simulink model "sim_battery_system"  (R2018b)
settings: Solver=FixedStepDiscrete  StartTime=0.0  StopTime=SimPara.t_sim  FixedStep=SimPara.t_step  RelTol=1e-3
undefined symbols (not defined in the file or in its folder): A, BatPara, i, LSAPara, p, SimPara, SysPara, x2_cal, x3_cal, x_cal
libraries: simulink x14, dspstat3 x4, dspindex x1
(part 2 of 4)

== system sim_battery_system/Battery system simulation/Thermal Submodel/Cell heat transport and heat dissipation ==
  PQ_cell : Inport
  BatPara : Inport  Port=2
  T_cell_in : Inport  Port=3
  alpha_cell_ambient : Inport  Port=4
  T_cell_ambient : Inport  Port=5
  Enable : EnablePort
  Heat dissipation model : Subsystem
  Heat transfer between cells : Subsystem  Variant=on
  Lumped mass thermal cell model : Subsystem  VariantControl=SimPara.heat_exchange_enable == 0
  T_cell [°C] : Outport  InitialOutput=SysPara.BatStateInit.thermal.T_cell
  PQ_ambient [W] : Outport  Port=2  InitialOutput=0
  PQ_transfer [W] : Outport  Port=3  InitialOutput=0
  wires:
  Lumped mass thermal cell model/1(T_cell [°C]) -> T_cell [°C]/1
  PQ_cell/1 -> Lumped mass thermal cell model/1(PQ_cell)
  BatPara/1 -> Heat dissipation model/2(BatPara), Lumped mass thermal cell model/2(BatPara)
  T_cell_in/1 -> Heat transfer between cells/1(T_cell_in), Heat dissipation model/1(T_cells_in), Lumped mass thermal cell model/3(T_cell_in)
  T_cell_ambient/1 -> Heat dissipation model/3(T_cell_ambient)
  alpha_cell_ambient/1 -> Heat dissipation model/4(alpha_cell_ambient)
  Heat dissipation model/1(PQ_ambient) -> PQ_ambient [W]/1, Lumped mass thermal cell model/4(PQ_ambient)
  Heat transfer between cells/1(PQ_transfer) -> PQ_transfer [W]/1, Lumped mass thermal cell model/5(PQ_transfer)

== system sim_battery_system/Battery system simulation/Thermal Submodel/Irreversible heat generation ==
  note: Calculation of ohmic/irreversible heat losses:
      |
      | -> Equation PQ_Cells,irr = R_Cells,total * I_Cells^2
      | -> R_Cells is the sum of all voltage drops in the cell (internal resistance and RC-Elements)
  U_R [V] : Inport
  U_RC : Inport  Port=2
  I_Cells [A] : Inport  Port=3
  Abs : Abs
  Add : Sum
  Bus Selector : BusSelector  OutputSignals=sum_U_RC [V]
  Product : Product  Inputs=**  RndMeth=Zero
  PQ_cell,irr [W] : Outport
  wires:
  I_Cells [A]/1 -> Product/2
  Add/1 -> Product/1
  Product/1 -> Abs/1
  U_R [V]/1 -> Add/1
  U_RC/1 -> Bus Selector/1
  Abs/1 -> PQ_cell,irr [W]/1  "PQ_cell,irr"
  Bus Selector/1 -> Add/2  "<sum_U_RC [V]>"

== system sim_battery_system/Battery system simulation/Thermal Submodel/Reversible heat generation ==
  note: Calculation of reversible heat losses in the cells
      |
      | PQ_Cells,rev = - I_cell * T_cell * (dUocv/dT_cell) = - I_cell * T_cell * EnCo
      |
      | Eddahech et al., 2013 - Thermal characterization of a high-power lithium-ion battery
  I_Cells [A] : Inport
  T_Cells [°C] : Inport  Port=2
  BatPara : Inport  Port=3
  Bus Selector : BusSelector  OutputSignals=thermal.EnCo
  Gain : Gain  Gain=-1
  Product : Product  Inputs=***  RndMeth=Zero
  PQ_cell,rev [W] : Outport
  wires:
  BatPara/1 -> Bus Selector/1
  Product/1 -> Gain/1
  T_Cells [°C]/1 -> Product/3
  I_Cells [A]/1 -> Product/1
  Gain/1 -> PQ_cell,rev [W]/1  "PQ_cell,rev"
  Bus Selector/1 -> Product/2  "<EnCo>"

== system sim_battery_system/Monitoring and Logging/Load Spectrum Analysis/Load Spectrum Analysis OFF ==
  BatState_el : Inport
  BatState_th : Inport  Port=2
  BatPara : Inport  Port=3
  Terminator : Terminator
  Terminator1 : Terminator
  Terminator2 : Terminator
  wires:
  BatState_el/1 -> Terminator/1
  BatState_th/1 -> Terminator1/1
  BatPara/1 -> Terminator2/1

== system sim_battery_system/Monitoring and Logging/Load Spectrum Analysis/Load Spectrum Analysis ON ==
  BatState_el : Inport
  BatState_th : Inport  Port=2
  BatPara : Inport  Port=3
  Bus Selector : BusSelector  OutputSignals=SOC,I_cell [A],U_cell [V]
  Bus Selector1 : BusSelector  OutputSignals=T_cell [°C]
  Bus Selector2 : BusSelector  OutputSignals=electrical.C_A [Ah]
  Load Spectrum Analysis ON : Subsystem  VariantControl=SimPara.LoadSpectra == 1
  wires:
  BatState_el/1 -> Bus Selector/1
  BatState_th/1 -> Bus Selector1/1
  BatPara/1 -> Bus Selector2/1
  Bus Selector/1 -> Load Spectrum Analysis ON/1(SOC)  "<SOC>"
  Bus Selector/2 -> Load Spectrum Analysis ON/2(I_cell [A])  "<I_cell [A]>"
  Bus Selector/3 -> Load Spectrum Analysis ON/3(U_Cell [A])  "<U_cell [V]>"
  Bus Selector1/1 -> Load Spectrum Analysis ON/4(T_cell [°C])  "<T_cell [°C]>"
  Bus Selector2/1 -> Load Spectrum Analysis ON/5(C_A [Ah])  "<C_A [Ah]>"

== system sim_battery_system/Monitoring and Logging/Logging of Variables/Calc Temp Gradient ==
  T_cell : Inport
  Abs : Abs
  Add : Sum  Inputs=-+
  MinMax : MinMax
  MinMax1 : MinMax  Function=max
  Reshape : Reshape
  T_cell_gradient : Outport
  wires:
  T_cell/1 -> Reshape/1
  MinMax/1 -> Add/1
  MinMax1/1 -> Add/2
  Add/1 -> Abs/1
  Abs/1 -> T_cell_gradient/1
  Reshape/1 -> MinMax1/1, MinMax/1

== system sim_battery_system/Monitoring and Logging/Temperature Sensor Simulation/Enable//disable temperature sensors ==
  T_cell : Inport
  TempSensors OFF : Subsystem  VariantControl=SimPara.TempSensors_enable==0
  TempSensors ON : Subsystem  VariantControl=SimPara.TempSensors_enable==1
  T_sensors [°C] : Outport

== system sim_battery_system/Monitoring and Logging/Temperature Sensor Simulation/Rebuild bus structure ==
  T_sensors : Inport
  Bat_state_th_in : Inport  Port=2
  Bus Creator1 : BusCreator  Inputs=7
  Bus Selector1 : BusSelector  OutputSignals=PQ_cell [W],T_cell [°C],T_cell_ambient,alpha_cell_ambient,PQ_ambient [W],PQ_transfer [W]
  bat_state_th_out : Outport
  wires:
  Bus Selector1/4 -> Bus Creator1/4  "<alpha_cell_ambient>"
  Bus Selector1/1 -> Bus Creator1/1  "<PQ_cell [W]>"
  Bus Selector1/2 -> Bus Creator1/2  "<T_cell [°C]>"
  T_sensors/1 -> Bus Creator1/7
  Bus Selector1/3 -> Bus Creator1/3  "<T_cell_ambient>"
  Bat_state_th_in/1 -> Bus Selector1/1
  Bus Creator1/1 -> bat_state_th_out/1  "bat_state_th"
  Bus Selector1/5 -> Bus Creator1/5  "<PQ_ambient [W]>"
  Bus Selector1/6 -> Bus Creator1/6  "<PQ_transfer [W]>"

== system sim_battery_system/Battery system simulation/Electrical Submodel/Electric potential (single cell)/Cell ECM RC-element 1 ==
  BatState_In : Inport
  BatPara : Inport  Port=2
  dt [s] : Inport  Port=3
  Enable : EnablePort
  Bus Selector : BusSelector  OutputSignals=U_RC.U_RC1 [V],I_cell [A]
  Bus Selector1 : BusSelector  OutputSignals=electrical.R1 [Ohm],electrical.C1 [F]
  Constant : Constant  VectorParams1D=off
  Gain : Gain  Gain=-1
  Math Function : Math  SaturateOnIntegerOverflow=on
  Product : Product  Inputs=**  RndMeth=Zero
  Product1 : Product  Inputs=/*  RndMeth=Zero
  Product2 : Product  Inputs=***  RndMeth=Zero
  Product3 : Product  Inputs=**  RndMeth=Zero
  Sum : Sum  Inputs=-+
  Sum1 : Sum
  U_RC1 [V] : Outport  OutputWhenDisabled=reset  InitialOutput=zeros(SysPara.p,SysPara.s)
  wires:
  Product/1 -> Product1/1
  Product3/1 -> Sum1/1
  Product1/1 -> Gain/1
  Sum1/1 -> U_RC1 [V]/1
  Gain/1 -> Math Function/1
  Product2/1 -> Sum1/2
  Bus Selector/1 -> Product3/1  "<U_RC1 [V]>"
  Math Function/1 -> Sum/1, Product3/2
  Sum/1 -> Product2/1
  Bus Selector1/1 -> Product2/2, Product/1  "<R1 [Ohm]>"
  BatPara/1 -> Bus Selector1/1
  dt [s]/1 -> Product1/2
  Bus Selector/2 -> Product2/3  "<I_cell [A]>"
  BatState_In/1 -> Bus Selector/1
  Bus Selector1/2 -> Product/2  "<C1 [F]>"
  Constant/1 -> Sum/2

== system sim_battery_system/Battery system simulation/Electrical Submodel/Electric potential (single cell)/Cell ECM RC-element 2 ==
  BatState_In : Inport
  BatPara : Inport  Port=2
  dt [s] : Inport  Port=3
  Enable : EnablePort
  Bus Selector : BusSelector  OutputSignals=U_RC.U_RC2 [V],I_cell [A]
  Bus Selector1 : BusSelector  OutputSignals=electrical.R2 [Ohm],electrical.C2 [F]
  Constant : Constant  VectorParams1D=off
  Gain : Gain  Gain=-1
  Math Function : Math  SaturateOnIntegerOverflow=on
  Product : Product  Inputs=**  RndMeth=Zero
  Product1 : Product  Inputs=/*  RndMeth=Zero
  Product2 : Product  Inputs=***  RndMeth=Zero
  Product3 : Product  Inputs=**  RndMeth=Zero
  Sum : Sum  Inputs=-+
  Sum1 : Sum
  U_RC2 [V] : Outport  OutputWhenDisabled=reset  InitialOutput=zeros(SysPara.p,SysPara.s)
  wires:
  Product/1 -> Product1/1
  Product3/1 -> Sum1/1
  Product1/1 -> Gain/1
  Sum1/1 -> U_RC2 [V]/1
  Gain/1 -> Math Function/1
  Product2/1 -> Sum1/2
  Bus Selector/1 -> Product3/1  "<U_RC2 [V]>"
  Math Function/1 -> Sum/1, Product3/2
  Sum/1 -> Product2/1
  Bus Selector1/1 -> Product2/2, Product/1  "<R2 [Ohm]>"
  BatPara/1 -> Bus Selector1/1
  dt [s]/1 -> Product1/2
  Bus Selector/2 -> Product2/3  "<I_cell [A]>"
  BatState_In/1 -> Bus Selector/1
  Bus Selector1/2 -> Product/2  "<C2 [F]>"
  Constant/1 -> Sum/2

== system sim_battery_system/Battery system simulation/Electrical Submodel/Electric potential (single cell)/Cell ECM RC-element 3 ==
  BatState_In : Inport
  BatPara : Inport  Port=2
  dt [s] : Inport  Port=3
  Enable : EnablePort
  Bus Selector : BusSelector  OutputSignals=U_RC.U_RC3 [V],I_cell [A]
  Bus Selector1 : BusSelector  OutputSignals=electrical.R3 [Ohm],electrical.C3 [F]
  Constant : Constant  VectorParams1D=off
  Gain : Gain  Gain=-1
  Math Function : Math  SaturateOnIntegerOverflow=on
  Product : Product  Inputs=**  RndMeth=Zero
  Product1 : Product  Inputs=/*  RndMeth=Zero
  Product2 : Product  Inputs=***  RndMeth=Zero
  Product3 : Product  Inputs=**  RndMeth=Zero
  Sum : Sum  Inputs=-+
  Sum1 : Sum
  U_RC3 [V] : Outport  OutputWhenDisabled=reset  InitialOutput=zeros(SysPara.p,SysPara.s)
  wires:
  Product/1 -> Product1/1
  Product3/1 -> Sum1/1
  Product1/1 -> Gain/1
  Sum1/1 -> U_RC3 [V]/1
  Gain/1 -> Math Function/1
  Product2/1 -> Sum1/2
  Bus Selector/1 -> Product3/1  "<U_RC3 [V]>"
  Math Function/1 -> Sum/1, Product3/2
  Sum/1 -> Product2/1
  Bus Selector1/1 -> Product2/2, Product/1  "<R3 [Ohm]>"
  BatPara/1 -> Bus Selector1/1
  dt [s]/1 -> Product1/2
  Bus Selector/2 -> Product2/3  "<I_cell [A]>"
  BatState_In/1 -> Bus Selector/1
  Bus Selector1/2 -> Product/2  "<C3 [F]>"
  Constant/1 -> Sum/2

== system sim_battery_system/Battery system simulation/Electrical Submodel/Electric potential (single cell)/Cell ECM RC-element 4 ==
  BatState_In : Inport
  BatPara : Inport  Port=2
  dt [s] : Inport  Port=3
  Enable : EnablePort
  Bus Selector : BusSelector  OutputSignals=U_RC.U_RC4 [V],I_cell [A]
  Bus Selector1 : BusSelector  OutputSignals=electrical.R4 [Ohm],electrical.C4 [F]
  Constant : Constant  VectorParams1D=off
  Gain : Gain  Gain=-1
  Math Function : Math  SaturateOnIntegerOverflow=on
  Product : Product  Inputs=**  RndMeth=Zero
  Product1 : Product  Inputs=/*  RndMeth=Zero
  Product2 : Product  Inputs=***  RndMeth=Zero
  Product3 : Product  Inputs=**  RndMeth=Zero
  Sum : Sum  Inputs=-+
  Sum1 : Sum
  U_RC4 [V] : Outport  OutputWhenDisabled=reset  InitialOutput=zeros(SysPara.p,SysPara.s)
  wires:
  Product/1 -> Product1/1
  Product3/1 -> Sum1/1
  Product1/1 -> Gain/1
  Sum1/1 -> U_RC4 [V]/1
  Gain/1 -> Math Function/1
  Product2/1 -> Sum1/2
  Bus Selector/1 -> Product3/1  "<U_RC4 [V]>"
  Math Function/1 -> Sum/1, Product3/2
  Sum/1 -> Product2/1
  Bus Selector1/1 -> Product2/2, Product/1  "<R4 [Ohm]>"
  BatPara/1 -> Bus Selector1/1
  dt [s]/1 -> Product1/2
  Bus Selector/2 -> Product2/3  "<I_cell [A]>"
  BatState_In/1 -> Bus Selector/1
  Bus Selector1/2 -> Product/2  "<C4 [F]>"
  Constant/1 -> Sum/2

== system sim_battery_system/Battery system simulation/Electrical Submodel/Electric potential (single cell)/Cell Hysteresis Voltage ==
  note: Zugrunde liegende Formel aus "Verbrugge, 2007 - Adaptive, multi-parameter battery state estimator with optimized time weighting factors"
  note: Wenn kein Hysteresemodell verwendet werden soll
      |  beta = 0 setzen
  BatState_In : Inport
  dt [s] : Inport  Port=2
  Add : Sum  Inputs=-+
  Add1 : Sum
  Bus Selector : BusSelector  OutputSignals=U_Hysteresis [V],I_cell [A],SOC
  Product : Product
  Product1 : Product  Inputs=4
  Sign : Signum
  V_H,max(SOC) : Lookup_n-D  NumberOfTableDimensions=1  BreakpointsForDimension1=BatPara.electrical.OCV.SOC  BeginIndexSearchUsingPreviousIndexResult=on  Table=BatPara.electrical.OCV.U_hyst  ExtrapMethod=Clip  DiagnosticForOutOfRangeInput=Warning  RemoveProtectionInput=on  UseLastTableValue=on  InternalRulePriority=Speed  RndMeth=Simplest  InputSameDT=on
  beta : Constant  Value=BatPara.electrical.OCV.beta_hyst  VectorParams1D=off
  U_Hysteresis [V] : Outport
  wires:
  Bus Selector/2 -> Sign/1, Product1/3  "<I_cell [A]>"
  Bus Selector/3 -> V_H,max(SOC)/1  "<SOC>"
  V_H,max(SOC)/1 -> Add/2
  Add/1 -> Product1/4  "V_H,max-sign(I)*V_H"
  dt [s]/1 -> Product1/2
  Product1/1 -> Add1/2
  Add1/1 -> U_Hysteresis [V]/1
  Sign/1 -> Product/2  "sign(I)"
  Product/1 -> Add/1
  BatState_In/1 -> Bus Selector/1
  Bus Selector/1 -> Add1/1, Product/1  "<U_Hysteresis [V]>"
  beta/1 -> Product1/1

== system sim_battery_system/Battery system simulation/Electrical Submodel/Electric potential (single cell)/Cell Open-Circuit-Voltage ==
  SOC [-] : Inport
  BatPara : Inport  Port=2
  SOC --> U : Lookup_n-D  NumberOfTableDimensions=1  BreakpointsForDimension1=BatPara.electrical.OCV.SOC  BreakpointsForDimension2=[1:3]  IndexSearchMethod=Linear search  BeginIndexSearchUsingPreviousIndexResult=on  Table=BatPara.electrical.OCV.U  DiagnosticForOutOfRangeInput=Warning  RemoveProtectionInput=on  RndMeth=Simplest  InputSameDT=on
  Terminator : Terminator
  U_OCV [V] : Outport
  wires:
  SOC [-]/1 -> SOC --> U/1
  SOC --> U/1 -> U_OCV [V]/1
  BatPara/1 -> Terminator/1

== system sim_battery_system/Battery system simulation/Electrical Submodel/Electric potential (single cell)/Cell SOC ==
  BatPara : Inport
  BatState_In : Inport  Port=2
  dt [s] : Inport  Port=3
  Ah in As : Gain  Gain=3600
  Bus Selector : BusSelector  OutputSignals=electrical.C_A [Ah]
  Bus Selector1 : BusSelector  OutputSignals=I_cell [A],SOC
  Product : Product  Inputs=**/  RndMeth=Zero
  Sum : Sum
  SOC [-] : Outport
  wires:
  Bus Selector1/2 -> Sum/2  "<SOC>"
  Product/1 -> Sum/1  "delta_SOC"
  Bus Selector/1 -> Ah in As/1  "<C_A [Ah]>"
  Ah in As/1 -> Product/3
  Bus Selector1/1 -> Product/2  "<I_cell [A]>"
  dt [s]/1 -> Product/1
  BatState_In/1 -> Bus Selector1/1
  BatPara/1 -> Bus Selector/1
  Sum/1 -> SOC [-]/1

== system sim_battery_system/Battery system simulation/Thermal Submodel/Cell heat transport and heat dissipation/Heat dissipation model ==
  note: Determination of the heat fluxes between the cells and their environments:
      | à No heat exchange between adjacent cells in the battery pack (optionally done in subsystem 'Heat transfer between cells')
      | à Each individual cell is independently viewed and has its own environmental temperature and heat transfer coefficient to the environment (defined by model input 'BTMS_input' at the top level of the model).
      | à Heat flow between a cell and its environment only via convection
      | PQ_Ambient* = alpha_cell_mbient * A * (T_cell_ambient - T_cell*)
  T_cells_in : Inport
  BatPara : Inport  Port=2
  T_cell_ambient : Inport  Port=3
  alpha_cell_ambient : Inport  Port=4
  Bus Selector2 : BusSelector  OutputSignals=physical.A [m^2]
  Product : Product  Inputs=3
  Subtract : Sum  Inputs=+-
  PQ_ambient : Outport
  wires:
  Bus Selector2/1 -> Product/2  "<A [m^2]>"
  T_cells_in/1 -> Subtract/2
  Subtract/1 -> Product/3
  BatPara/1 -> Bus Selector2/1
  T_cell_ambient/1 -> Subtract/1
  Product/1 -> PQ_ambient/1  "PQ_ambient [W]"
  alpha_cell_ambient/1 -> Product/1

== system sim_battery_system/Battery system simulation/Thermal Submodel/Cell heat transport and heat dissipation/Heat transfer between cells ==
  note: Variants:
      |
      | - Heat transfer model switched OFF: No heat transfer between cells, PQ_transfer is always 0
      |
      | - Heat transfer model switched OFF: Heat transfer between cells is simulated and a heat flux from/to every cell is computed.
  T_cell_in : Inport
  Heat transfer model switched OFF : Subsystem  VariantControl=SimPara.heat_exchange_enable == 0
  Heat transfer model switched ON : Subsystem  VariantControl=SimPara.heat_exchange_enable == 1
  PQ_transfer : Outport  InitialOutput=SysPara.BatStateInit.thermal.T_cell

== system sim_battery_system/Battery system simulation/Thermal Submodel/Cell heat transport and heat dissipation/Lumped mass thermal cell model ==
  note: Determination of the heat outputs which allow a temperature change of the cells:
      | à Sum of the individual heat outputs or flows for each cell
      | à The "Unit Delay" allows the heat outputs of the cells to be viewed from the previous evaluation time.
      | à By subtracting the temperatures of the cells from their ambient temperatures, the heat flows between the cells and their environments are properly defined for the equation
      | PQ_Temperature = PQ_cells + PQ_ambient + PQ_transfer
  note: Determination of the quantities of heat that allow the temperature of the cells to change:
      | à Heat quantity is integral of the heat output over time.
      | à Assumption that the heat outputs, which enable a temperature change of the cells, remain constant from the previous evaluation time until the current evaluation time.
      | à dt is time difference between two evaluations
      | Q_Temperature = PQ_Temperature* * dt
  note: Determination of the cell temperatures at the current evaluation time:
      | à Q_Temperature result in current temperature changes of the cells compared to the previous evaluation time.
      | Q_Temperature = m * c * (T_cell - T_cell*)
      | à T_cell = Q_Temperature / (m * c) + T_cell*
  PQ_cell : Inport
  BatPara : Inport  Port=2
  T_cell_in : Inport  Port=3
  PQ_ambient : Inport  Port=4
  PQ_transfer : Inport  Port=5
  Add1 : Sum
  Bus Selector1 : BusSelector  OutputSignals=physical.m [kg],thermal.c [J/(kg*K)]
  Divide : Product  Inputs=*/
  Product1 : Product
  Product2 : Product
  Subtract1 : Sum  Inputs=+++
  dt : Subsystem
  T_cell [°C] : Outport
  wires:
  T_cell_in/1 -> Add1/2
  BatPara/1 -> Bus Selector1/1
  PQ_cell/1 -> Subtract1/1
  Bus Selector1/1 -> Product2/1  "<m [kg]>"
  Bus Selector1/2 -> Product2/2  "<c [J/(kg*K)]>"
  Subtract1/1 -> Product1/2  "PQ_Temperature"
  dt/1(dt [s]) -> Product1/1
  Divide/1 -> Add1/1
  Product2/1 -> Divide/2
  Add1/1 -> T_cell [°C]/1  "T_cell [°C]"
  Product1/1 -> Divide/1  "Q_Temperature"
  PQ_ambient/1 -> Subtract1/2
  PQ_transfer/1 -> Subtract1/3

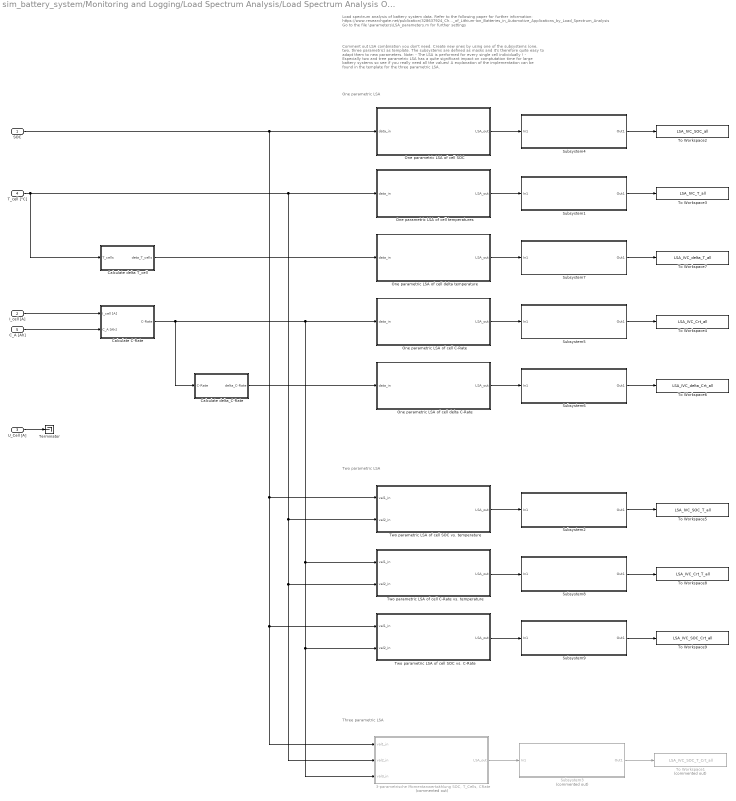
== system sim_battery_system/Monitoring and Logging/Load Spectrum Analysis/Load Spectrum Analysis ON/Load Spectrum Analysis ON ==
  note: Comment out LSA combination you don't need. Create new ones by using one of the subsystems (one, two, three parametric) as template. The subsystems are defined as masks
      | and it's therefore quite easy to adapt them to new parameters.
      |
      | Note:
      | - The LSA is performed for every single cell individually !
      | - Especially two and tree parametric LSA has a quite significant impact on comptutation time for large battery systems so see if you really need all the values!
      |
      | A explanation of the implementation can be found in the template for the three parametric LSA.
  note: Three parametric LSA
  note: Two parametric LSA
  note: One parametric LSA
  note: Load spectrum analysis of battery system data. Refer to the following paper for further information:
      | https://www.researchgate.net/publication/328637924_Characterization_and_Concept_Validation_of_Lithium-Ion_Batteries_in_Automotive_Applications_by_Load_Spectrum_Analysis
      |
      | Go to the file \parameters\LSA_parameters.m for further settings
  SOC : Inport
  I_cell [A] : Inport  Port=2
  U_Cell [A] : Inport  Port=3
  T_cell [°C] : Inport  Port=4
  C_A [Ah] : Inport  Port=5
  "3-parametrische Momentanwertzählung SOC, T_Cells, CRate" : Subsystem  Commented=on  mask{bins_borders_1=LSAPara.bins_borders_SOC, bins_mean_1=LSAPara.bins_mean_SOC, bins_borders_2=LSAPara.bins_borders_T, bins_mean_2=LSAPara.bins_mean_T, bins_borders_3=LSAPara.bins_borders_Crt, bins_mean_3=LSAPara.bins_mean_Crt}
      mask prompts: bins_borders_1 "Provide 'bins_borders'"; bins_mean_1 "Provide 'bins_mean'"; bins_borders_2 "Provide 'bins_borders'"; bins_mean_2 "Provide 'bins_mean'"; bins_borders_3 "Provide 'bins_borders'"; bins_mean_3 "Provide 'bins_mean'"
      mask DialogControl DescTextVar Prompt: Subsystem for three-parametric instantaneous value counting. Change the parameters below to select other system variables. Refer to parameters\LSA_parameters.m for further options.
      mask DialogControl Control2 Prompt: Copy&Paste this subsystem and double click to edit the variable assignments to monitor further variables.
      mask DialogControl Control3 Prompt: First system variable ('val 1')
      mask DialogControl Control4 Prompt: First system variable ('val 2')
      mask DialogControl Control5 Prompt: First system variable ('val 3')
      mask Display:
      | fprintf('Three parametric\ninstantaneous value\ncounting')
      | port_label('output', 1, 'load spectrum')
      | port_label('input', 1, 'timeseries val 1')
      | port_label('input', 2, 'timeseries val 2')
      | port_label('input', 3, 'timeseries val 3')
  Calculate C-Rate : Subsystem
  Calculate delta T_cell : Subsystem
  Calculate delta_C-Rate : Subsystem
  One parametric LSA of cell C-Rate : Subsystem  mask{bins_borders=LSAPara.bins_borders_Crt, bins_mean=LSAPara.bins_mean_Crt}
      mask prompts: bins_borders "Provide 'bins_borders'"; bins_mean "Provide 'bins_mean'"
      mask DialogControl DescTextVar Prompt: Subsystem for one-parametric instantaneous value counting. Change the parameters below to select other system variables. Refer to parameters\LSA_parameters.m for further options.
      mask DialogControl Control2 Prompt: Copy&Paste this subsystem and double click to edit the variable assignments to monitor further variables.
      mask Display:
      | fprintf('One parametric\ninstantaneous value\ncounting')
      | port_label('output', 1, 'load spectrum')
      | port_label('input', 1, 'timeseries')
  One parametric LSA of cell SOC : Subsystem  mask{bins_borders=LSAPara.bins_borders_SOC, bins_mean=LSAPara.bins_mean_SOC}
      mask prompts: bins_borders "Provide 'bins_borders'"; bins_mean "Provide 'bins_mean'"
      mask DialogControl DescTextVar Prompt: Subsystem for one-parametric instantaneous value counting. Change the parameters below to select other system variables. Refer to parameters\LSA_parameters.m for further options.
      mask DialogControl Control2 Prompt: Copy&Paste this subsystem and double click to edit the variable assignments to monitor further variables.
      mask Display:
      | fprintf('One parametric\ninstantaneous value\ncounting')
      | port_label('output', 1, 'load spectrum')
      | port_label('input', 1, 'timeseries')
  One parametric LSA of cell delta C-Rate : Subsystem  mask{bins_borders=LSAPara.bins_borders_delta_Crt, bins_mean=LSAPara.bins_mean_delta_Crt}
      mask prompts: bins_borders "Provide 'bins_borders'"; bins_mean "Provide 'bins_mean'"
      mask DialogControl DescTextVar Prompt: Subsystem for one-parametric instantaneous value counting. Change the parameters below to select other system variables. Refer to parameters\LSA_parameters.m for further options.
      mask DialogControl Control2 Prompt: Copy&Paste this subsystem and double click to edit the variable assignments to monitor further variables.
      mask Display:
      | fprintf('One parametric\ninstantaneous value\ncounting')
      | port_label('output', 1, 'load spectrum')
      | port_label('input', 1, 'timeseries')
  One parametric LSA of cell delta temperature : Subsystem  mask{bins_borders=LSAPara.bins_borders_delta_T, bins_mean=LSAPara.bins_mean_delta_T}
      mask prompts: bins_borders "Provide 'bins_borders'"; bins_mean "Provide 'bins_mean'"
      mask DialogControl DescTextVar Prompt: Subsystem for one-parametric instantaneous value counting. Change the parameters below to select other system variables. Refer to parameters\LSA_parameters.m for further options.
      mask DialogControl Control2 Prompt: Copy&Paste this subsystem and double click to edit the variable assignments to monitor further variables.
      mask Display:
      | fprintf('One parametric\ninstantaneous value\ncounting')
      | port_label('output', 1, 'load spectrum')
      | port_label('input', 1, 'timeseries')
  One parametric LSA of cell temperatures : Subsystem  mask{bins_borders=LSAPara.bins_borders_T, bins_mean=LSAPara.bins_mean_T}
      mask prompts: bins_borders "Provide 'bins_borders'"; bins_mean "Provide 'bins_mean'"
      mask DialogControl DescTextVar Prompt: Subsystem for one-parametric instantaneous value counting. Change the parameters below to select other system variables. Refer to parameters\LSA_parameters.m for further options.
      mask DialogControl Control2 Prompt: Copy&Paste this subsystem and double click to edit the variable assignments to monitor further variables.
      mask Display:
      | fprintf('One parametric\ninstantaneous value\ncounting')
      | port_label('output', 1, 'load spectrum')
      | port_label('input', 1, 'timeseries')
  Subsystem1 : Subsystem  mask{dim=2, start=99}
      mask prompts: dim "Select dimension"; start "Start concatenation after x%"
      mask DialogControl DescTextVar Prompt: Create one load spectrum from all individual cells. By default the LSA blocks create one load spectrum for every individual cell. This block creates one load-spectrum for all cells.
      mask DialogControl Control2 Prompt: Select the dimension of the load spectum in the parameter below. This uses the following logic:
      mask DialogControl Control3 Prompt: One parametric LS: Select "2"
      mask DialogControl Control4 Prompt: Two parametric LS: Select "3"
      mask DialogControl Control5 Prompt: Three parametric LS: Select "4"
      mask DialogControl Control6 Prompt: Only the last value of the load spectrum matrix is relevant, so we don't want to make the concatenation every simulation step. Therefore the system is set to only start with the calculation after 99% of the simulation is finished. If you need another value edit ist below.
      mask Display:
      | fprintf('Summed LSA\nfrom all cells')
      | port_label('input', 1, 'cell-individual LSA')
      | port_label('output', 1, 'summed LSA')
  Subsystem2 : Subsystem  mask{dim=3, start=99}
      mask prompts: dim "Select dimension"; start "Start concatenation after x%"
      mask DialogControl DescTextVar Prompt: Create one load spectrum from all individual cells. By default the LSA blocks create one load spectrum for every individual cell. This block creates one load-spectrum for all cells.
      mask DialogControl Control2 Prompt: Select the dimension of the load spectum in the parameter below. This uses the following logic:
      mask DialogControl Control3 Prompt: One parametric LS: Select "2"
      mask DialogControl Control4 Prompt: Two parametric LS: Select "3"
      mask DialogControl Control5 Prompt: Three parametric LS: Select "4"
      mask DialogControl Control6 Prompt: Only the last value of the load spectrum matrix is relevant, so we don't want to make the concatenation every simulation step. Therefore the system is set to only start with the calculation after 99% of the simulation is finished. If you need another value edit ist below.
      mask Display:
      | fprintf('Summed LSA\nfrom all cells')
      | port_label('input', 1, 'cell-individual LSA')
      | port_label('output', 1, 'summed LSA')
  Subsystem3 : Subsystem  Commented=on  mask{dim=4, start=99}
      mask prompts: dim "Select dimension"; start "Start concatenation after x%"
      mask DialogControl DescTextVar Prompt: Create one load spectrum from all individual cells. By default the LSA blocks create one load spectrum for every individual cell. This block creates one load-spectrum for all cells.
      mask DialogControl Control2 Prompt: Select the dimension of the load spectum in the parameter below. This uses the following logic:
      mask DialogControl Control3 Prompt: One parametric LS: Select "2"
      mask DialogControl Control4 Prompt: Two parametric LS: Select "3"
      mask DialogControl Control5 Prompt: Three parametric LS: Select "4"
      mask DialogControl Control6 Prompt: Only the last value of the load spectrum matrix is relevant, so we don't want to make the concatenation every simulation step. Therefore the system is set to only start with the calculation after 99% of the simulation is finished. If you need another value edit ist below.
      mask Display:
      | fprintf('Summed LSA\nfrom all cells')
      | port_label('input', 1, 'cell-individual LSA')
      | port_label('output', 1, 'summed LSA')
  Subsystem4 : Subsystem  mask{dim=2, start=99}
      mask prompts: dim "Select dimension"; start "Start concatenation after x%"
      mask DialogControl DescTextVar Prompt: Create one load spectrum from all individual cells. By default the LSA blocks create one load spectrum for every individual cell. This block creates one load-spectrum for all cells.
      mask DialogControl Control2 Prompt: Select the dimension of the load spectum in the parameter below. This uses the following logic:
      mask DialogControl Control3 Prompt: One parametric LS: Select "2"
      mask DialogControl Control4 Prompt: Two parametric LS: Select "3"
      mask DialogControl Control5 Prompt: Three parametric LS: Select "4"
      mask DialogControl Control6 Prompt: Only the last value of the load spectrum matrix is relevant, so we don't want to make the concatenation every simulation step. Therefore the system is set to only start with the calculation after 99% of the simulation is finished. If you need another value edit ist below.
      mask Display:
      | fprintf('Summed LSA\nfrom all cells')
      | port_label('input', 1, 'cell-individual LSA')
      | port_label('output', 1, 'summed LSA')
  Subsystem5 : Subsystem  mask{dim=2, start=99}
      mask prompts: dim "Select dimension"; start "Start concatenation after x%"
      mask DialogControl DescTextVar Prompt: Create one load spectrum from all individual cells. By default the LSA blocks create one load spectrum for every individual cell. This block creates one load-spectrum for all cells.
      mask DialogControl Control2 Prompt: Select the dimension of the load spectum in the parameter below. This uses the following logic:
      mask DialogControl Control3 Prompt: One parametric LS: Select "2"
      mask DialogControl Control4 Prompt: Two parametric LS: Select "3"
      mask DialogControl Control5 Prompt: Three parametric LS: Select "4"
      mask DialogControl Control6 Prompt: Only the last value of the load spectrum matrix is relevant, so we don't want to make the concatenation every simulation step. Therefore the system is set to only start with the calculation after 99% of the simulation is finished. If you need another value edit ist below.
      mask Display:
      | fprintf('Summed LSA\nfrom all cells')
      | port_label('input', 1, 'cell-individual LSA')
      | port_label('output', 1, 'summed LSA')
  Subsystem6 : Subsystem  mask{dim=2, start=99}
      mask prompts: dim "Select dimension"; start "Start concatenation after x%"
      mask DialogControl DescTextVar Prompt: Create one load spectrum from all individual cells. By default the LSA blocks create one load spectrum for every individual cell. This block creates one load-spectrum for all cells.
      mask DialogControl Control2 Prompt: Select the dimension of the load spectum in the parameter below. This uses the following logic:
      mask DialogControl Control3 Prompt: One parametric LS: Select "2"
      mask DialogControl Control4 Prompt: Two parametric LS: Select "3"
      mask DialogControl Control5 Prompt: Three parametric LS: Select "4"
      mask DialogControl Control6 Prompt: Only the last value of the load spectrum matrix is relevant, so we don't want to make the concatenation every simulation step. Therefore the system is set to only start with the calculation after 99% of the simulation is finished. If you need another value edit ist below.
      mask Display:
      | fprintf('Summed LSA\nfrom all cells')
      | port_label('input', 1, 'cell-individual LSA')
      | port_label('output', 1, 'summed LSA')
  Subsystem7 : Subsystem  mask{dim=2, start=99}
      mask prompts: dim "Select dimension"; start "Start concatenation after x%"
      mask DialogControl DescTextVar Prompt: Create one load spectrum from all individual cells. By default the LSA blocks create one load spectrum for every individual cell. This block creates one load-spectrum for all cells.
      mask DialogControl Control2 Prompt: Select the dimension of the load spectum in the parameter below. This uses the following logic:
      mask DialogControl Control3 Prompt: One parametric LS: Select "2"
      mask DialogControl Control4 Prompt: Two parametric LS: Select "3"
      mask DialogControl Control5 Prompt: Three parametric LS: Select "4"
      mask DialogControl Control6 Prompt: Only the last value of the load spectrum matrix is relevant, so we don't want to make the concatenation every simulation step. Therefore the system is set to only start with the calculation after 99% of the simulation is finished. If you need another value edit ist below.
      mask Display:
      | fprintf('Summed LSA\nfrom all cells')
      | port_label('input', 1, 'cell-individual LSA')
      | port_label('output', 1, 'summed LSA')
  Subsystem8 : Subsystem  mask{dim=3, start=99}
      mask prompts: dim "Select dimension"; start "Start concatenation after x%"
      mask DialogControl DescTextVar Prompt: Create one load spectrum from all individual cells. By default the LSA blocks create one load spectrum for every individual cell. This block creates one load-spectrum for all cells.
      mask DialogControl Control2 Prompt: Select the dimension of the load spectum in the parameter below. This uses the following logic:
      mask DialogControl Control3 Prompt: One parametric LS: Select "2"
      mask DialogControl Control4 Prompt: Two parametric LS: Select "3"
      mask DialogControl Control5 Prompt: Three parametric LS: Select "4"
      mask DialogControl Control6 Prompt: Only the last value of the load spectrum matrix is relevant, so we don't want to make the concatenation every simulation step. Therefore the system is set to only start with the calculation after 99% of the simulation is finished. If you need another value edit ist below.
      mask Display:
      | fprintf('Summed LSA\nfrom all cells')
      | port_label('input', 1, 'cell-individual LSA')
      | port_label('output', 1, 'summed LSA')
  Subsystem9 : Subsystem  mask{dim=3, start=99}
      mask prompts: dim "Select dimension"; start "Start concatenation after x%"
      mask DialogControl DescTextVar Prompt: Create one load spectrum from all individual cells. By default the LSA blocks create one load spectrum for every individual cell. This block creates one load-spectrum for all cells.
      mask DialogControl Control2 Prompt: Select the dimension of the load spectum in the parameter below. This uses the following logic:
      mask DialogControl Control3 Prompt: One parametric LS: Select "2"
      mask DialogControl Control4 Prompt: Two parametric LS: Select "3"
      mask DialogControl Control5 Prompt: Three parametric LS: Select "4"
      mask DialogControl Control6 Prompt: Only the last value of the load spectrum matrix is relevant, so we don't want to make the concatenation every simulation step. Therefore the system is set to only start with the calculation after 99% of the simulation is finished. If you need another value edit ist below.
      mask Display:
      | fprintf('Summed LSA\nfrom all cells')
      | port_label('input', 1, 'cell-individual LSA')
      | port_label('output', 1, 'summed LSA')
  Terminator : Terminator
  To Workspace1 : ToWorkspace  Commented=on  VariableName=LSA_IVC_SOC_T_Crt_all  SampleTime=-1
      settings: MaxDataPoints=1
  To Workspace2 : ToWorkspace  VariableName=LSA_IVC_SOC_all  SampleTime=-1
      settings: MaxDataPoints=1
  To Workspace3 : ToWorkspace  VariableName=LSA_IVC_T_all  SampleTime=-1
      settings: MaxDataPoints=1
  To Workspace4 : ToWorkspace  VariableName=LSA_IVC_Crt_all  SampleTime=-1
      settings: MaxDataPoints=1
  To Workspace5 : ToWorkspace  VariableName=LSA_IVC_SOC_T_all  SampleTime=-1
      settings: MaxDataPoints=1
  To Workspace6 : ToWorkspace  VariableName=LSA_IVC_delta_Crt_all  SampleTime=-1
      settings: MaxDataPoints=1
  To Workspace7 : ToWorkspace  VariableName=LSA_IVC_delta_T_all  SampleTime=-1
      settings: MaxDataPoints=1
  To Workspace8 : ToWorkspace  VariableName=LSA_IVC_Crt_T_all  SampleTime=-1
      settings: MaxDataPoints=1
  To Workspace9 : ToWorkspace  VariableName=LSA_IVC_SOC_Crt_all  SampleTime=-1
      settings: MaxDataPoints=1
  Two parametric LSA of cell C-Rate vs. temperature : Subsystem  mask{bins_borders_1=LSAPara.bins_borders_Crt, bins_mean_1=LSAPara.bins_mean_Crt, bins_borders_2=LSAPara.bins_borders_T, bins_mean_2=LSAPara.bins_mean_T}
      mask prompts: bins_borders_1 "Provide 'bins_borders'"; bins_mean_1 "Provide 'bins_mean'"; bins_borders_2 "Provide 'bins_borders'"; bins_mean_2 "Provide 'bins_mean'"
      mask DialogControl DescTextVar Prompt: Subsystem for twp-parametric instantaneous value counting. Change the parameters below to select other system variables. Refer to parameters\LSA_parameters.m for further options.
      mask DialogControl Control2 Prompt: Copy&Paste this subsystem and double click to edit the variable assignments to monitor further variables.
      mask DialogControl Control3 Prompt: First system variable ('val 1')
      mask DialogControl Control4 Prompt: Second system variable ('val 2')
      mask Display:
      | fprintf('Two parametric\ninstantaneous value\ncounting')
      | port_label('output', 1, 'load spectrum')
      | port_label('input', 1, 'timeseries val 1')
      | port_label('input', 2, 'timeseries val 2')
  Two parametric LSA of cell SOC vs. C-Rate : Subsystem  mask{bins_borders_1=LSAPara.bins_borders_SOC, bins_mean_1=LSAPara.bins_mean_SOC, bins_borders_2=LSAPara.bins_borders_Crt, bins_mean_2=LSAPara.bins_mean_Crt}
      mask prompts: bins_borders_1 "Provide 'bins_borders'"; bins_mean_1 "Provide 'bins_mean'"; bins_borders_2 "Provide 'bins_borders'"; bins_mean_2 "Provide 'bins_mean'"
      mask DialogControl DescTextVar Prompt: Subsystem for twp-parametric instantaneous value counting. Change the parameters below to select other system variables. Refer to parameters\LSA_parameters.m for further options.
      mask DialogControl Control2 Prompt: Copy&Paste this subsystem and double click to edit the variable assignments to monitor further variables.
      mask DialogControl Control3 Prompt: First system variable ('val 1')
      mask DialogControl Control4 Prompt: Second system variable ('val 2')
      mask Display:
      | fprintf('Two parametric\ninstantaneous value\ncounting')
      | port_label('output', 1, 'load spectrum')
      | port_label('input', 1, 'timeseries val 1')
      | port_label('input', 2, 'timeseries val 2')
  "Two parametric LSA of cell SOC vs. temperature " : Subsystem  mask{bins_borders_1=LSAPara.bins_borders_SOC, bins_mean_1=LSAPara.bins_mean_SOC, bins_borders_2=LSAPara.bins_borders_T, bins_mean_2=LSAPara.bins_mean_T}
      mask prompts: bins_borders_1 "Provide 'bins_borders'"; bins_mean_1 "Provide 'bins_mean'"; bins_borders_2 "Provide 'bins_borders'"; bins_mean_2 "Provide 'bins_mean'"
      mask DialogControl DescTextVar Prompt: Subsystem for twp-parametric instantaneous value counting. Change the parameters below to select other system variables. Refer to parameters\LSA_parameters.m for further options.
      mask DialogControl Control2 Prompt: Copy&Paste this subsystem and double click to edit the variable assignments to monitor further variables.
      mask DialogControl Control3 Prompt: First system variable ('val 1')
      mask DialogControl Control4 Prompt: Second system variable ('val 2')
      mask Display:
      | fprintf('Two parametric\ninstantaneous value\ncounting')
      | port_label('output', 1, 'load spectrum')
      | port_label('input', 1, 'timeseries val 1')
      | port_label('input', 2, 'timeseries val 2')
  wires:
  I_cell [A]/1 -> Calculate C-Rate/1(I_cell [A])
  SOC/1 -> "3-parametrische Momentanwertzählung SOC, T_Cells, CRate"/1(val1_in), Two parametric LSA of cell SOC vs. C-Rate/1(val1_in), "Two parametric LSA of cell SOC vs. temperature "/1(val1_in), One parametric LSA of cell SOC/1(data_in)
  C_A [Ah]/1 -> Calculate C-Rate/2(C_A [Ah])
  Calculate C-Rate/1(C-Rate) -> Calculate delta_C-Rate/1(C-Rate), One parametric LSA of cell C-Rate/1(data_in), "3-parametrische Momentanwertzählung SOC, T_Cells, CRate"/3(val3_in), Two parametric LSA of cell SOC vs. C-Rate/2(val2_in), Two parametric LSA of cell C-Rate vs. temperature/1(val1_in)
  "3-parametrische Momentanwertzählung SOC, T_Cells, CRate"/1(LSA_out) -> Subsystem3/1(In1)
  Subsystem1/1(Out1) -> To Workspace3/1
  One parametric LSA of cell temperatures/1(LSA_out) -> Subsystem1/1(In1)
  "Two parametric LSA of cell SOC vs. temperature "/1(LSA_out) -> Subsystem2/1(In1)
  Subsystem2/1(Out1) -> To Workspace5/1
  Subsystem3/1(Out1) -> To Workspace1/1
  U_Cell [A]/1 -> Terminator/1
  Calculate delta_C-Rate/1(delta_C-Rate) -> One parametric LSA of cell delta C-Rate/1(data_in)
  T_cell [°C]/1 -> Calculate delta T_cell/1(T_cells), One parametric LSA of cell temperatures/1(data_in), "3-parametrische Momentanwertzählung SOC, T_Cells, CRate"/2(val2_in), Two parametric LSA of cell C-Rate vs. temperature/2(val2_in), "Two parametric LSA of cell SOC vs. temperature "/2(val2_in)
  Calculate delta T_cell/1(deta_T_cells) -> One parametric LSA of cell delta temperature/1(data_in)
  Subsystem4/1(Out1) -> To Workspace2/1
  Subsystem5/1(Out1) -> To Workspace4/1
  Subsystem6/1(Out1) -> To Workspace6/1
  Subsystem7/1(Out1) -> To Workspace7/1
  One parametric LSA of cell SOC/1(LSA_out) -> Subsystem4/1(In1)
  One parametric LSA of cell C-Rate/1(LSA_out) -> Subsystem5/1(In1)
  One parametric LSA of cell delta C-Rate/1(LSA_out) -> Subsystem6/1(In1)
  One parametric LSA of cell delta temperature/1(LSA_out) -> Subsystem7/1(In1)
  Subsystem8/1(Out1) -> To Workspace8/1
  Subsystem9/1(Out1) -> To Workspace9/1
  Two parametric LSA of cell C-Rate vs. temperature/1(LSA_out) -> Subsystem8/1(In1)
  Two parametric LSA of cell SOC vs. C-Rate/1(LSA_out) -> Subsystem9/1(In1)

== system sim_battery_system/Monitoring and Logging/Temperature Sensor Simulation/Enable//disable temperature sensors/TempSensors OFF ==
  T_cell : Inport
  Constant : Constant  Value=0  OutDataTypeStr=boolean
  Terminator : Terminator
  T_sensors [°C] : Outport
  wires:
  T_cell/1 -> Terminator/1
  Constant/1 -> T_sensors [°C]/1  "T_sensors [°C]"

== system sim_battery_system/Monitoring and Logging/Temperature Sensor Simulation/Enable//disable temperature sensors/TempSensors ON ==
  T_cell : Inport
  Iterate through the sensors : Subsystem  TreatAsAtomicUnit=on
  Matrix to vector : Reshape  OutputDimensionality=Column vector (2-D)
  T_sensors [°C] : Outport
  wires:
  Matrix to vector/1 -> Iterate through the sensors/1(T_cells_vec)
  T_cell/1 -> Matrix to vector/1
  Iterate through the sensors/1(T_sensors [°C]) -> T_sensors [°C]/1  "T_sensors [°C]"

== system sim_battery_system/Battery system simulation/Thermal Submodel/Cell heat transport and heat dissipation/Heat transfer between cells/Heat transfer model switched OFF ==
  note: Heat transfer model switched off.
      | No heat transfer.
  T_cell_in : Inport
  Constant : Constant  Value=0
  Terminator1 : Terminator
  PQ_transfer : Outport
  wires:
  T_cell_in/1 -> Terminator1/1
  Constant/1 -> PQ_transfer/1  "PQ_transfer [W]"

== system sim_battery_system/Battery system simulation/Thermal Submodel/Cell heat transport and heat dissipation/Heat transfer between cells/Heat transfer model switched ON ==
  note: Calculate the heat transfer between cells:
      | - Cells exchange heat via a heat transfer coefficient.
      | - Those are defined in the matrix K_transfer
      | -Example for cell 1 exchanging heat will cell i:
      | PQ_lambda_cell = sum((T_i-T_1)/K_transfer(i,1))
  note: PQ_lambda = K_transfer * T_cell_in
  note: Column vector --> Matrix
  note: Matrix --> column vector
  T_cell_in : Inport
  Constant : Constant  Value=SysPara.thermal.transfer.K_transfer
  Product : Product  Multiplication=Matrix(*)
  Reshape1 : Reshape  OutputDimensionality=Column vector (2-D)
  Reshape2 : Reshape  OutputDimensionality=Customize  OutputDimensions=[SysPara.p, SysPara.s]
  PQ_transfer : Outport
  wires:
  T_cell_in/1 -> Reshape1/1
  Reshape2/1 -> PQ_transfer/1  "PQ_transfer [W]"
  Reshape1/1 -> Product/2
  Product/1 -> Reshape2/1
  Constant/1 -> Product/1

== system sim_battery_system/Battery system simulation/Thermal Submodel/Cell heat transport and heat dissipation/Lumped mass thermal cell model/dt ==
  Clock : Clock
  Subtract : Sum  Inputs=+-
  Unit Delay : UnitDelay  SampleTime=-1
  dt [s] : Outport
  wires:
  Unit Delay/1 -> Subtract/2
  Clock/1 -> Unit Delay/1, Subtract/1
  Subtract/1 -> dt [s]/1

== system sim_battery_system/Monitoring and Logging/Load Spectrum Analysis/Load Spectrum Analysis ON/Load Spectrum Analysis ON/3-parametrische Momentanwertzählung SOC, T_Cells, CRate ==
  val1_in : Inport
  val2_in : Inport  Port=2
  val3_in : Inport  Port=3
  For Iterator val1 : Subsystem  TreatAsAtomicUnit=on
  delay for selector data input : UnitDelay  SampleTime=-1
  LSA_out : Outport
  wires:
  val3_in/1 -> For Iterator val1/3(val3_in)
  val2_in/1 -> For Iterator val1/2(val2_in)
  val1_in/1 -> For Iterator val1/1(val1_in)
  For Iterator val1/1(LSA_out) -> LSA_out/1, delay for selector data input/1
  delay for selector data input/1 -> For Iterator val1/4(data_in_delayed)

== system sim_battery_system/Monitoring and Logging/Load Spectrum Analysis/Load Spectrum Analysis ON/Load Spectrum Analysis ON/Calculate C-Rate ==
  note: Note: We calculate the C-Rate for each cell using each cell's individual C_A!
  I_cell [A] : Inport
  C_A [Ah] : Inport  Port=2
  I --> C-Rate : Product  Inputs=*/
  C-Rate : Outport
  wires:
  I --> C-Rate/1 -> C-Rate/1
  I_cell [A]/1 -> I --> C-Rate/1
  C_A [Ah]/1 -> I --> C-Rate/2

== system sim_battery_system/Monitoring and Logging/Load Spectrum Analysis/Load Spectrum Analysis ON/Load Spectrum Analysis ON/Calculate delta T_cell ==
  T_cells : Inport
  Add : Sum  Inputs=+-
  Minimum : dspstat3/Minimum  operation=minimum  fcn=Value  indexBase=One  operateOver=Entire input  Dimension=1  InputProcessing=Columns as channels (frame based)  reset=None  roiEnable=off  roiType=Rectangles  roiPortion=Entire ROI  roiOutput=Individual statistics for each ROI  roiFlag=off  roundingMode=Floor  overflowMode=off
      settings: SourceProductName=DSP System Toolbox  SourceProductBaseCode=DS
  deta_T_cells : Outport
  wires:
  T_cells/1 -> Add/1, Minimum/1
  Add/1 -> deta_T_cells/1
  Minimum/1 -> Add/2

== system sim_battery_system/Monitoring and Logging/Load Spectrum Analysis/Load Spectrum Analysis ON/Load Spectrum Analysis ON/Calculate delta_C-Rate ==
  note: Calculate the delta_C-Rate for each cell in respect to the lowest absolute C-Rate in the system for each time-step.
  C-Rate : Inport
  Bildung Differenz : Sum  Inputs=+-
  Minimum1 : dspstat3/Minimum  operation=minimum  fcn=Value  indexBase=One  operateOver=Entire input  Dimension=1  InputProcessing=Columns as channels (frame based)  reset=None  roiEnable=off  roiType=Rectangles  roiPortion=Entire ROI  roiOutput=Individual statistics for each ROI  roiFlag=off  roundingMode=Floor  overflowMode=off
      settings: SourceProductName=DSP System Toolbox  SourceProductBaseCode=DS
  Product : Product
  Sign : Signum
  always positve : Abs
  delta_C-Rate : Outport
  wires:
  always positve/1 -> Minimum1/1
  Bildung Differenz/1 -> delta_C-Rate/1
  Sign/1 -> Product/1
  C-Rate/1 -> Bildung Differenz/1, Sign/1, always positve/1
  Minimum1/1 -> Product/2
  Product/1 -> Bildung Differenz/2

== system sim_battery_system/Monitoring and Logging/Load Spectrum Analysis/Load Spectrum Analysis ON/Load Spectrum Analysis ON/One parametric LSA of cell C-Rate ==
  data_in : Inport
  For Iterator val1 : Subsystem  TreatAsAtomicUnit=on
  delay for selector data input : UnitDelay  SampleTime=-1
  LSA_out : Outport
  wires:
  data_in/1 -> For Iterator val1/1(data_in)
  For Iterator val1/1(LSA_out) -> delay for selector data input/1, LSA_out/1
  delay for selector data input/1 -> For Iterator val1/2(data_in_delay)

== system sim_battery_system/Monitoring and Logging/Load Spectrum Analysis/Load Spectrum Analysis ON/Load Spectrum Analysis ON/One parametric LSA of cell SOC ==
  data_in : Inport
  For Iterator val1 : Subsystem  TreatAsAtomicUnit=on
  delay for selector data input : UnitDelay  SampleTime=-1
  LSA_out : Outport
  wires:
  delay for selector data input/1 -> For Iterator val1/2(data_in_delay)
  For Iterator val1/1(LSA_out) -> LSA_out/1, delay for selector data input/1
  data_in/1 -> For Iterator val1/1(data_in)

== system sim_battery_system/Monitoring and Logging/Load Spectrum Analysis/Load Spectrum Analysis ON/Load Spectrum Analysis ON/One parametric LSA of cell delta C-Rate ==
  data_in : Inport
  For Iterator val1 : Subsystem  TreatAsAtomicUnit=on
  delay for selector data input : UnitDelay  SampleTime=-1
  LSA_out : Outport
  wires:
  delay for selector data input/1 -> For Iterator val1/2(data_in_delay)
  For Iterator val1/1(LSA_out) -> LSA_out/1, delay for selector data input/1
  data_in/1 -> For Iterator val1/1(data_in)
